simulink model "controlGPI_pos_6dof_sinMI"  (R2023b)
settings: Solver=ode45  StartTime=0.0  StopTime=tsim  FixedStep=tstep  MaxStep=tstep  RelTol=tstep/10
undefined symbols (not defined in the file): contr_robot_params, ddq, dq, ndof, NN_Bspline_params, NN_RBF_params, nn_select, Pc, q0, q_cero, q_eq, robot_params, t_qeq_init, t_tr_init, t_trtr, tau_L, tau_L_mags, tr_muestra, tr_ref, Wc, Zc
libraries: simulink x2
(part 2 of 2)

== system controlGPI_pos_6dof_sinMI/Trayectoria de referencia/3 to 9 (4) ==
  In1 : Inport
  In2 : Inport  Port=2
  In3 : Inport  Port=3
  Demux2 : Demux  Outputs=3
  Demux3 : Demux  Outputs=3
  Demux4 : Demux  Outputs=3
  Out1 : Outport
  Out2 : Outport  Port=2
  Out3 : Outport  Port=3
  Out4 : Outport  Port=4
  Out5 : Outport  Port=5
  Out6 : Outport  Port=6
  Out7 : Outport  Port=7
  Out8 : Outport  Port=8
  Out9 : Outport  Port=9
  wires:
  In3/1 -> Demux4/1
  Demux4/1 -> Out3/1
  Demux2/1 -> Out1/1
  Demux3/3 -> Out8/1
  Demux3/2 -> Out5/1
  Demux3/1 -> Out2/1
  In1/1 -> Demux2/1
  Demux2/3 -> Out7/1
  Demux4/3 -> Out9/1
  Demux4/2 -> Out6/1
  Demux2/2 -> Out4/1
  In2/1 -> Demux3/1

== system controlGPI_pos_6dof_sinMI/Trayectoria de referencia/3 to 9 (5) ==
  In1 : Inport
  In2 : Inport  Port=2
  In3 : Inport  Port=3
  Demux2 : Demux  Outputs=3
  Demux3 : Demux  Outputs=3
  Demux4 : Demux  Outputs=3
  Out1 : Outport
  Out2 : Outport  Port=2
  Out3 : Outport  Port=3
  Out4 : Outport  Port=4
  Out5 : Outport  Port=5
  Out6 : Outport  Port=6
  Out7 : Outport  Port=7
  Out8 : Outport  Port=8
  Out9 : Outport  Port=9
  wires:
  In3/1 -> Demux4/1
  Demux4/1 -> Out3/1
  Demux2/1 -> Out1/1
  Demux3/3 -> Out8/1
  Demux3/2 -> Out5/1
  Demux3/1 -> Out2/1
  In1/1 -> Demux2/1
  Demux2/3 -> Out7/1
  Demux4/3 -> Out9/1
  Demux4/2 -> Out6/1
  Demux2/2 -> Out4/1
  In2/1 -> Demux3/1

== system controlGPI_pos_6dof_sinMI/Trayectoria de referencia/3 to 9 (7) ==
  In1 : Inport
  In2 : Inport  Port=2
  In3 : Inport  Port=3
  Demux2 : Demux  Outputs=3
  Demux3 : Demux  Outputs=3
  Demux4 : Demux  Outputs=3
  Out1 : Outport
  Out2 : Outport  Port=2
  Out3 : Outport  Port=3
  Out4 : Outport  Port=4
  Out5 : Outport  Port=5
  Out6 : Outport  Port=6
  Out7 : Outport  Port=7
  Out8 : Outport  Port=8
  Out9 : Outport  Port=9
  wires:
  In3/1 -> Demux4/1
  Demux4/1 -> Out3/1
  Demux2/1 -> Out1/1
  Demux3/3 -> Out8/1
  Demux3/2 -> Out5/1
  Demux3/1 -> Out2/1
  In1/1 -> Demux2/1
  Demux2/3 -> Out7/1
  Demux4/3 -> Out9/1
  Demux4/2 -> Out6/1
  Demux2/2 -> Out4/1
  In2/1 -> Demux3/1

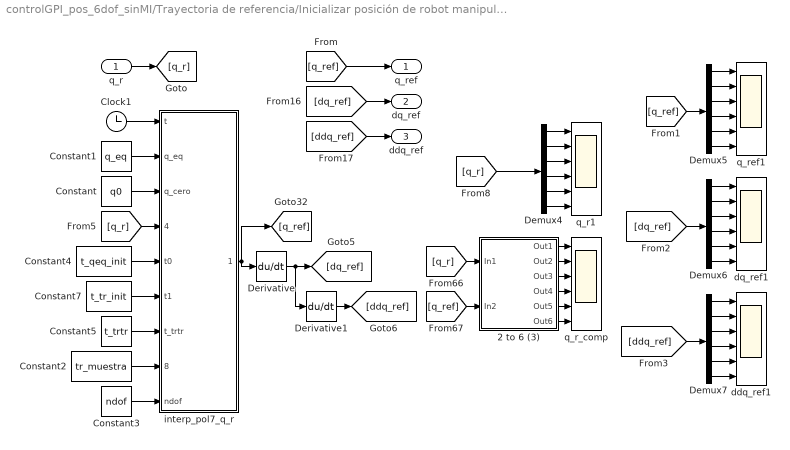
== system controlGPI_pos_6dof_sinMI/Trayectoria de referencia/Inicializar posición de robot manipulador ==
  q_r : Inport
  2 to 6 (3) : Subsystem
  Clock1 : Clock
  Constant : Constant  Value=q0
  Constant1 : Constant  Value=q_eq
  Constant2 : Constant  Value=tr_muestra
  Constant3 : Constant  Value=ndof
  Constant4 : Constant  Value=t_qeq_init
  Constant5 : Constant  Value=t_trtr
  Constant7 : Constant  Value=t_tr_init
  Demux{4..7} (4 alike) : Demux  Outputs=6
  Derivative : Derivative
  Derivative1 : Derivative
  ddq_ref1 : Scope  NumInputPorts=6
  dq_ref1 : Scope  NumInputPorts=6
  interp_pol7_q_r : MATLAB Function  TreatAsAtomicUnit=on
  q_r1 : Scope  NumInputPorts=6
  q_r_comp : Scope  NumInputPorts=6
  q_ref1 : Scope  NumInputPorts=6
  q_ref : Outport
  dq_ref : Outport  Port=2
  ddq_ref : Outport  Port=3
  wires:
  [ddq_ref] -> ddq_ref/1
  q_r/1 -> [q_r]
  [dq_ref] -> dq_ref/1
  [q_ref] -> q_ref/1
  2 to 6 (3)/1(Out1) -> q_r_comp/1
  [q_r] -> 2 to 6 (3)/1(In1)
  2 to 6 (3)/3(Out3) -> q_r_comp/3
  2 to 6 (3)/5(Out5) -> q_r_comp/5
  2 to 6 (3)/6(Out6) -> q_r_comp/6
  [q_ref] -> 2 to 6 (3)/2(In2)
  2 to 6 (3)/2(Out2) -> q_r_comp/2
  2 to 6 (3)/4(Out4) -> q_r_comp/4
  Demux4/3 -> q_r1/3
  Demux4/5 -> q_r1/5
  Demux4/4 -> q_r1/4
  Demux4/2 -> q_r1/2
  Demux4/6 -> q_r1/6
  Demux4/1 -> q_r1/1
  [q_r] -> Demux4/1
  Constant7/1 -> interp_pol7_q_r/6(t1)
  Clock1/1 -> interp_pol7_q_r/1(t)
  interp_pol7_q_r/1(interp_qpos) -> Derivative/1, [q_ref]
  Constant1/1 -> interp_pol7_q_r/2(q_eq)
  Constant/1 -> interp_pol7_q_r/3(q_cero)
  Derivative/1 -> [dq_ref], Derivative1/1
  Derivative1/1 -> [ddq_ref]
  Demux5/6 -> q_ref1/6
  Demux5/2 -> q_ref1/2
  [q_ref] -> Demux5/1
  Demux5/1 -> q_ref1/1
  Demux5/4 -> q_ref1/4
  Demux5/5 -> q_ref1/5
  Demux5/3 -> q_ref1/3
  Demux6/1 -> dq_ref1/1
  Demux6/4 -> dq_ref1/4
  Demux6/5 -> dq_ref1/5
  [dq_ref] -> Demux6/1
  Demux6/6 -> dq_ref1/6
  Demux6/2 -> dq_ref1/2
  Demux6/3 -> dq_ref1/3
  Demux7/2 -> ddq_ref1/2
  Demux7/4 -> ddq_ref1/4
  Demux7/3 -> ddq_ref1/3
  [ddq_ref] -> Demux7/1
  Demux7/1 -> ddq_ref1/1
  Demux7/6 -> ddq_ref1/6
  Demux7/5 -> ddq_ref1/5
  [q_r] -> interp_pol7_q_r/4(q_tr_init)
  Constant4/1 -> interp_pol7_q_r/5(t0)
  Constant2/1 -> interp_pol7_q_r/8(tr_muestra)
  Constant3/1 -> interp_pol7_q_r/9(ndof)
  Constant5/1 -> interp_pol7_q_r/7(t_trtr)

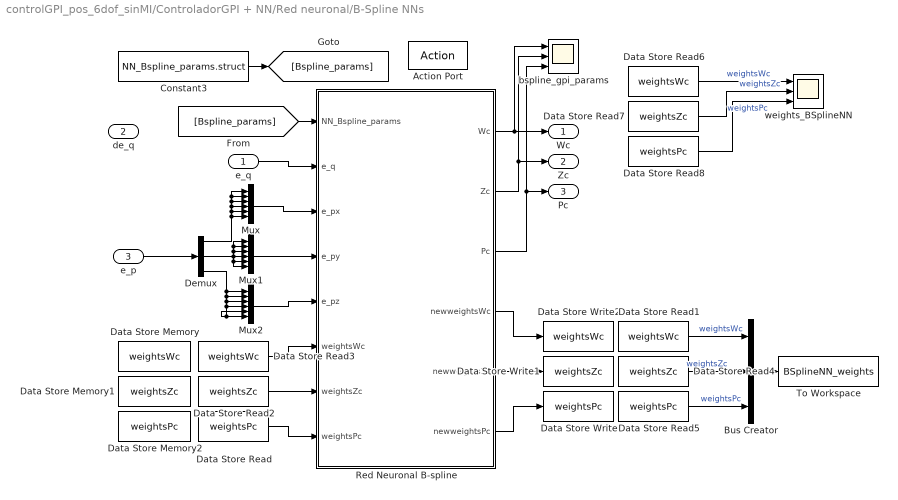
== system controlGPI_pos_6dof_sinMI/ControladorGPI + NN/Red neuronal/B-Spline NNs ==
  e_q : Inport
  de_q : Inport  Port=2
  e_p : Inport  Port=3
  Action Port : ActionPort  ActionPortLabel=if(u1 == 1)
  Bus Creator : BusCreator  Inputs=3
  Constant3 : Constant  Value=NN_Bspline_params.struct  OutDataTypeStr=Bus: NN_Bspline_params_bus
  Data Store Memory : DataStoreMemory  DataStoreName=weightsWc  WriteAfterWriteMsg=warning  InitialValue=NN_Bspline_params.weights.weightWc  ShowAdditionalParam=off  OutDataTypeStr=double
  Data Store Memory1 : DataStoreMemory  DataStoreName=weightsZc  WriteAfterWriteMsg=warning  InitialValue=NN_Bspline_params.weights.weightZc  ShowAdditionalParam=off  OutDataTypeStr=double
  Data Store Memory2 : DataStoreMemory  DataStoreName=weightsPc  WriteAfterWriteMsg=warning  InitialValue=NN_Bspline_params.weights.weightPc  ShowAdditionalParam=off  OutDataTypeStr=double
  Data Store Read : DataStoreRead  DataStoreName=weightsPc  IndexOptions=Index vector (dialog)  Indices=1  OutputSizes=1
  Data Store Read1 : DataStoreRead  DataStoreName=weightsWc  IndexOptions=Index vector (dialog)  Indices=1  OutputSizes=1
  Data Store Read2 : DataStoreRead  DataStoreName=weightsZc  IndexOptions=Index vector (dialog)  Indices=1  OutputSizes=1
  Data Store Read3 : DataStoreRead  DataStoreName=weightsWc  IndexOptions=Index vector (dialog)  Indices=1  OutputSizes=1
  Data Store Read4 : DataStoreRead  DataStoreName=weightsZc  IndexOptions=Index vector (dialog)  Indices=1  OutputSizes=1
  Data Store Read5 : DataStoreRead  DataStoreName=weightsPc  IndexOptions=Index vector (dialog)  Indices=1  OutputSizes=1
  Data Store Read6 : DataStoreRead  DataStoreName=weightsWc  IndexOptions=Index vector (dialog)  Indices=1  OutputSizes=1
  Data Store Read7 : DataStoreRead  DataStoreName=weightsZc  IndexOptions=Index vector (dialog)  Indices=1  OutputSizes=1
  Data Store Read8 : DataStoreRead  DataStoreName=weightsPc  IndexOptions=Index vector (dialog)  Indices=1  OutputSizes=1
  Data Store Write : DataStoreWrite  DataStoreName=weightsPc  IndexOptions=Index vector (dialog)  Indices=1  OutputSizes=1
  Data Store Write1 : DataStoreWrite  DataStoreName=weightsZc  IndexOptions=Index vector (dialog)  Indices=1  OutputSizes=1
  Data Store Write2 : DataStoreWrite  DataStoreName=weightsWc  IndexOptions=Index vector (dialog)  Indices=1  OutputSizes=1
  Demux : Demux  Outputs=3
  Mux : Mux  Inputs=6
  Mux1 : Mux  Inputs=6
  Mux2 : Mux  Inputs=6
  Red Neuronal B-spline : MATLAB Function  TreatAsAtomicUnit=on
  To Workspace : ToWorkspace  VariableName=BSplineNN_weights  SaveFormat=Timeseries  SampleTime=-1
  bspline_gpi_params : Scope  NumInputPorts=3
  weights_BSplineNN : Scope  NumInputPorts=3
  Wc : Outport
  Zc : Outport  Port=2
  Pc : Outport  Port=3
  wires:
  e_q/1 -> Red Neuronal B-spline/2(e_q)
  [Bspline_params] -> Red Neuronal B-spline/1(NN_Bspline_params)
  Red Neuronal B-spline/1(Wc) -> bspline_gpi_params/1, Wc/1
  Red Neuronal B-spline/2(Zc) -> bspline_gpi_params/2, Zc/1
  Red Neuronal B-spline/3(Pc) -> bspline_gpi_params/3, Pc/1
  Constant3/1 -> [Bspline_params]
  Data Store Read1/1 -> Bus Creator/1  "weightsWc"
  Data Store Read5/1 -> Bus Creator/3  "weightsPc"
  Bus Creator/1 -> To Workspace/1
  Data Store Read4/1 -> Bus Creator/2  "weightsZc"
  Red Neuronal B-spline/4(newweightsWc) -> Data Store Write2/1
  Red Neuronal B-spline/5(newweightsZc) -> Data Store Write1/1
  Red Neuronal B-spline/6(newweightsPc) -> Data Store Write/1
  Data Store Read3/1 -> Red Neuronal B-spline/6(weightsWc)
  Data Store Read2/1 -> Red Neuronal B-spline/7(weightsZc)
  Data Store Read/1 -> Red Neuronal B-spline/8(weightsPc)
  Data Store Read6/1 -> weights_BSplineNN/1  "weightsWc"
  Data Store Read7/1 -> weights_BSplineNN/2  "weightsZc"
  Data Store Read8/1 -> weights_BSplineNN/3  "weightsPc"
  e_p/1 -> Demux/1
  Demux/3 -> Mux2/3, Mux2/5, Mux2/6, Mux2/4, Mux2/2, Mux2/1
  Mux/1 -> Red Neuronal B-spline/3(e_px)
  Demux/1 -> Mux/6, Mux/5, Mux/4, Mux/3, Mux/1, Mux/2
  Mux2/1 -> Red Neuronal B-spline/5(e_pz)
  Demux/2 -> Mux1/6, Mux1/5, Mux1/4, Mux1/2, Mux1/1, Mux1/3
  Mux1/1 -> Red Neuronal B-spline/4(e_py)

== system controlGPI_pos_6dof_sinMI/ControladorGPI + NN/Red neuronal/Constants ==
  Action Port : ActionPort  ActionPortLabel=else
  Constant : Constant  Value=Wc
  Constant1 : Constant  Value=Zc
  Constant2 : Constant  Value=Pc
  Scope1 : Scope  NumInputPorts=3
  Wc : Outport
  Zc : Outport  Port=2
  Pc : Outport  Port=3
  wires:
  Constant/1 -> Wc/1, Scope1/1
  Constant2/1 -> Scope1/3, Pc/1
  Constant1/1 -> Zc/1, Scope1/2

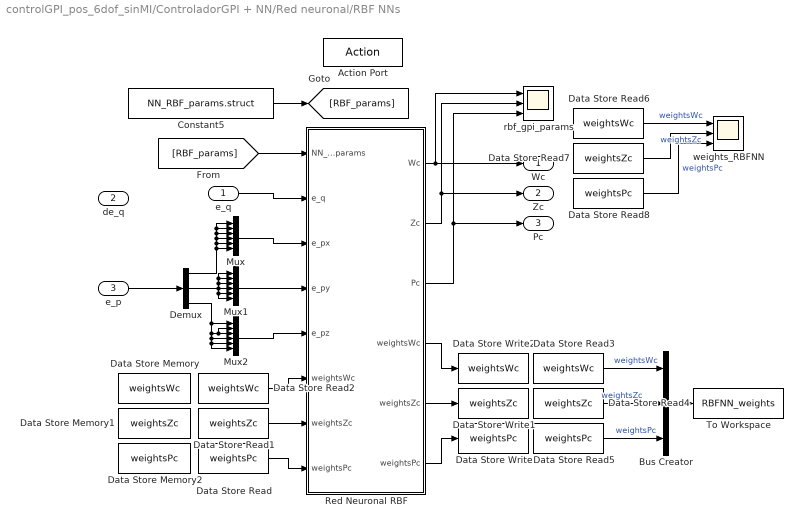
== system controlGPI_pos_6dof_sinMI/ControladorGPI + NN/Red neuronal/RBF NNs ==
  e_q : Inport
  de_q : Inport  Port=2
  e_p : Inport  Port=3
  Action Port : ActionPort  ActionPortLabel=elseif(u1 == 2)
  Bus Creator : BusCreator  Inputs=3
  Constant5 : Constant  Value=NN_RBF_params.struct  OutDataTypeStr=Bus: NN_RBF_params_bus
  Data Store Memory : DataStoreMemory  DataStoreName=weightsWc  WriteAfterWriteMsg=warning  InitialValue=NN_RBF_params.weights.weightWc  ShowAdditionalParam=off  OutDataTypeStr=double
  Data Store Memory1 : DataStoreMemory  DataStoreName=weightsZc  WriteAfterWriteMsg=warning  InitialValue=NN_RBF_params.weights.weightZc  ShowAdditionalParam=off  OutDataTypeStr=double
  Data Store Memory2 : DataStoreMemory  DataStoreName=weightsPc  WriteAfterWriteMsg=warning  InitialValue=NN_RBF_params.weights.weightPc  ShowAdditionalParam=off  OutDataTypeStr=double
  Data Store Read : DataStoreRead  DataStoreName=weightsPc  IndexOptions=Index vector (dialog)  Indices=1  OutputSizes=1
  Data Store Read1 : DataStoreRead  DataStoreName=weightsZc  IndexOptions=Index vector (dialog)  Indices=1  OutputSizes=1
  Data Store Read2 : DataStoreRead  DataStoreName=weightsWc  IndexOptions=Index vector (dialog)  Indices=1  OutputSizes=1
  Data Store Read3 : DataStoreRead  DataStoreName=weightsWc  IndexOptions=Index vector (dialog)  Indices=1  OutputSizes=1
  Data Store Read4 : DataStoreRead  DataStoreName=weightsZc  IndexOptions=Index vector (dialog)  Indices=1  OutputSizes=1
  Data Store Read5 : DataStoreRead  DataStoreName=weightsPc  IndexOptions=Index vector (dialog)  Indices=1  OutputSizes=1
  Data Store Read6 : DataStoreRead  DataStoreName=weightsWc  IndexOptions=Index vector (dialog)  Indices=1  OutputSizes=1
  Data Store Read7 : DataStoreRead  DataStoreName=weightsZc  IndexOptions=Index vector (dialog)  Indices=1  OutputSizes=1
  Data Store Read8 : DataStoreRead  DataStoreName=weightsPc  IndexOptions=Index vector (dialog)  Indices=1  OutputSizes=1
  Data Store Write : DataStoreWrite  DataStoreName=weightsPc  IndexOptions=Index vector (dialog)  Indices=1  OutputSizes=1
  Data Store Write1 : DataStoreWrite  DataStoreName=weightsZc  IndexOptions=Index vector (dialog)  Indices=1  OutputSizes=1
  Data Store Write2 : DataStoreWrite  DataStoreName=weightsWc  IndexOptions=Index vector (dialog)  Indices=1  OutputSizes=1
  Demux : Demux  Outputs=3
  Mux : Mux  Inputs=6
  Mux1 : Mux  Inputs=6
  Mux2 : Mux  Inputs=6
  Red Neuronal RBF : MATLAB Function  TreatAsAtomicUnit=on
  To Workspace : ToWorkspace  VariableName=RBFNN_weights  SaveFormat=Timeseries  SampleTime=-1
  rbf_gpi_params : Scope  NumInputPorts=3
  weights_RBFNN : Scope  NumInputPorts=3
  Wc : Outport
  Zc : Outport  Port=2
  Pc : Outport  Port=3
  wires:
  [RBF_params] -> Red Neuronal RBF/1(NN_RBF_params)
  e_q/1 -> Red Neuronal RBF/2(e_q)
  Red Neuronal RBF/1(Wc) -> rbf_gpi_params/1, Wc/1
  Red Neuronal RBF/2(Zc) -> rbf_gpi_params/2, Zc/1
  Red Neuronal RBF/3(Pc) -> rbf_gpi_params/3, Pc/1
  Data Store Read/1 -> Red Neuronal RBF/8("weightsPc ")
  Data Store Read1/1 -> Red Neuronal RBF/7("weightsZc ")
  Data Store Read2/1 -> Red Neuronal RBF/6("weightsWc ")
  Data Store Read3/1 -> Bus Creator/1  "weightsWc"
  Data Store Read4/1 -> Bus Creator/2  "weightsZc"
  Data Store Read5/1 -> Bus Creator/3  "weightsPc"
  Bus Creator/1 -> To Workspace/1
  Red Neuronal RBF/6(weightsPc) -> Data Store Write/1
  Red Neuronal RBF/4(weightsWc) -> Data Store Write2/1
  Red Neuronal RBF/5(weightsZc) -> Data Store Write1/1
  Data Store Read6/1 -> weights_RBFNN/1  "weightsWc"
  Data Store Read7/1 -> weights_RBFNN/2  "weightsZc"
  Data Store Read8/1 -> weights_RBFNN/3  "weightsPc"
  Constant5/1 -> [RBF_params]
  e_p/1 -> Demux/1
  Mux/1 -> Red Neuronal RBF/3(e_px)
  Mux1/1 -> Red Neuronal RBF/4(e_py)
  Demux/3 -> Mux2/6, Mux2/5, Mux2/4, Mux2/3, Mux2/2, Mux2/1
  Mux2/1 -> Red Neuronal RBF/5(e_pz)
  Demux/1 -> Mux/6, Mux/5, Mux/4, Mux/3, Mux/1, Mux/2
  Demux/2 -> Mux1/6, Mux1/5, Mux1/4, Mux1/2, Mux1/1, Mux1/3

== system controlGPI_pos_6dof_sinMI/Trayectoria de referencia/Inicializar posición de robot manipulador/2 to 6 (3) ==
  In1 : Inport
  In2 : Inport  Port=2
  Demux4 : Demux  Outputs=6
  Demux6 : Demux  Outputs=6
  Mux{,1..5} (6 alike) : Mux  Inputs=2
  Out1 : Outport
  Out2 : Outport  Port=2
  Out3 : Outport  Port=3
  Out4 : Outport  Port=4
  Out5 : Outport  Port=5
  Out6 : Outport  Port=6
  wires:
  In2/1 -> Demux6/1
  Demux4/3 -> Mux2/1
  Demux4/5 -> Mux4/1
  Demux4/6 -> Mux5/1
  Demux6/5 -> Mux4/2
  Demux4/1 -> Mux/1
  Demux6/6 -> Mux5/2
  In1/1 -> Demux4/1
  Demux4/4 -> Mux3/1
  Demux6/2 -> Mux1/2
  Demux6/4 -> Mux3/2
  Demux6/1 -> Mux/2
  Demux4/2 -> Mux1/1
  Demux6/3 -> Mux2/2
  Mux/1 -> Out1/1
  Mux1/1 -> Out2/1
  Mux2/1 -> Out3/1
  Mux3/1 -> Out4/1
  Mux4/1 -> Out5/1
  Mux5/1 -> Out6/1

== matlab function controlGPI_pos_6dof_sinMI/ControladorGPI + NN/Matriz de parámetros B ==
  data: B5 output size=[6,1]; B4 output size=[6,1]; B3 output size=[6,1]; B2 output size=[6,1]; Zc input size=[6,1]; B1 output size=[6,1]; Wc input size=[6,1]; Pc input size=[6,1]
function [B5,B4,B3,B2,B1] = fcn(Zc,Wc,Pc)

B = zeros(6,6);

B(:,1) = Wc.^4.*Pc;
B(:,2) = 4*Wc.^3.*Zc.*Pc + Wc.^4;
B(:,3) = 4*Wc.^3.*Zc + 4*Wc.^2.*Zc.^2.*Pc + 2.*Wc.^2.*Pc;
B(:,4) = 2*Wc.^2 + 4*Wc.^2.*Zc.^2 + 4*Wc.*Zc.*Pc;
B(:,5) = 4*Wc.*Zc + Pc;
% B(:,6) = ones(3,6);

B1 = B(:,1);
B2 = B(:,2);
B3 = B(:,3);
B4 = B(:,4);
B5 = B(:,5);
% B6 = B(:,6);

== matlab function controlGPI_pos_6dof_sinMI/ControladorGPI + NN/Red neuronal/B-Spline NNs/Red Neuronal B-spline ==
  data: NN_Bspline_params input; e_q input size=[6,1]; Wc output size=[6,1]; Zc output size=[6,1]; Pc output size=[6,1]; e_px input size=[6,1]; e_py input size=[6,1]; e_pz input size=[6,1]; newweightsWc output; newweightsZc output; newweightsPc output; weightsWc input; weightsZc input; weightsPc input
function [Wc, Zc, Pc, newweightsWc, newweightsZc, newweightsPc]   = BSpline_NN(NN_Bspline_params,e_q,e_px,e_py,e_pz,weightsWc,weightsZc,weightsPc)

deltaWc = NN_Bspline_params.delta.deltaWc;
deltaZc = NN_Bspline_params.delta.deltaZc;
deltaPc = NN_Bspline_params.delta.deltaPc;

lambdaWc = NN_Bspline_params.lambda.lambdaWc;
lambdaZc = NN_Bspline_params.lambda.lambdaZc;
lambdaPc = NN_Bspline_params.lambda.lambdaPc;

if NN_Bspline_params.num_inputs == 1
    nn_inputs = e_q;
elseif NN_Bspline_params.num_inputs == 4
    nn_inputs = [e_q,e_px,e_py,e_pz];
else
    nn_inputs = e_q;
end

delta = [deltaWc;
         deltaZc;
         deltaPc];

lambda = cat(1,lambdaWc,lambdaZc,lambdaPc);
weights = cat(1,weightsWc,weightsZc,weightsPc);

[newparams,newweights] = NN_Bspline.Gradient_Descent(delta,weights,lambda,nn_inputs);

Wc = newparams(1,:)';
Zc = newparams(2,:)';
Pc = newparams(3,:)';

newweightsWc = newweights(1,:,:);
newweightsZc = newweights(2,:,:);
newweightsPc = newweights(3,:,:);

end

== matlab function controlGPI_pos_6dof_sinMI/Perfil torque de carga tau_L/If Action Subsystem/Polinomio 7mo orden sen ==
  data: t input; perfil_params input; qpol output; vpol output; apol output; jpol output
function [qpol,vpol,apol,jpol] = fcn(t,perfil_params)

%Trayectoria de referencia

q0 = 0;
q1 = perfil_params.senoidal.amplitud;

% v0 = perfil_params.polinomio7.vel.inicial;
% v1 = perfil_params.polinomio7.vel.final;
% 
% ac0 = perfil_params.polinomio7.acel.inicial;
% ac1 = perfil_params.polinomio7.acel.final;
% 
% j0 = perfil_params.polinomio7.jerk.inicial;
% j1 = perfil_params.polinomio7.jerk.inicial;

if perfil_params.senoidal.tiempo_inicio-1>0
    t0 = perfil_params.senoidal.tiempo_inicio-1;
else
    t0 = 0;
end
t1 = perfil_params.senoidal.tiempo_inicio;

% Coeficientes de un polinomio de 7mo grado
[qpol,vpol,apol,jpol] = pol7(t,q1,q0,t0,t1);

== matlab function controlGPI_pos_6dof_sinMI/Perfil torque de carga tau_L/If Action Subsystem4/Polinomio 7mo orden tau_L ==
  data: t input; perfil_params input; qpol output; vpol output; apol output; jpol output
function [qpol,vpol,apol,jpol] = fcn(t,perfil_params)

%Trayectoria de referencia

q0 = perfil_params.polinomio7.pos.inicial;
q1 = perfil_params.polinomio7.pos.final;

% v0 = perfil_params.polinomio7.vel.inicial;
% v1 = perfil_params.polinomio7.vel.final;
% 
% ac0 = perfil_params.polinomio7.acel.inicial;
% ac1 = perfil_params.polinomio7.acel.final;
% 
% j0 = perfil_params.polinomio7.jerk.inicial;
% j1 = perfil_params.polinomio7.jerk.inicial;

t0 = perfil_params.polinomio7.tiempo.inicial;
t1 = perfil_params.polinomio7.tiempo.final;

% Coeficientes de un polinomio de 7mo grado
[qpol,vpol,apol,jpol] = pol7(t,q0,q1,t0,t1);

== matlab function controlGPI_pos_6dof_sinMI/Perfil torque de carga tau_L/If Action Subsystem7/Trayectoria 15 segmentos ==
  data: t input size=1; q output size=1; perfil_params input
function q = fcn(t,perfil_params)

q0 = perfil_params.tr15segs.pos.inicial;
q1 = perfil_params.tr15segs.pos.final;

t0 = perfil_params.tr15segs.tiempo.inicial;

vel_path = perfil_params.tr15segs.vel_path;
acel_path = perfil_params.tr15segs.acel_path;
snap_path = perfil_params.tr15segs.snap_path;

dist = norm(q1-q0);
num_steps = 1000;




[interq,T] = pol15segs.bounded_tr(dist,num_steps,vel_path,acel_path,snap_path,0);

tstep = T/num_steps;
t1 = t0 + T;
t_tr = (t0:tstep:t1)';


[~,idt] = min(t_tr-t);
dire = (q1 - q0)/dist;
q = q0 + dire*interq(idt);

== matlab function controlGPI_pos_6dof_sinMI/ISCI ==
  data: tau input; ISCI output
function ISCI = fcn(tau)

ISCI = tau.^2;

== matlab function controlGPI_pos_6dof_sinMI/Perfil torque de carga tau_L/If Action Subsystem6/Polinomio 7mo orden timeseries ==
  data: t input; qpol output; vpol output; apol output; jpol output
function [qpol,vpol,apol,jpol] = fcn(t)

q0 = 0;
q1 = 1;

t0 = 0.5;
t1 = 1;

%Trayectoria de referencia

% Coeficientes de un polinomio de 7mo grado
[qpol,vpol,apol,jpol] = pol7(t,q0,q1,t0,t1);

== matlab function controlGPI_pos_6dof_sinMI/Perfil torque de carga tau_L/If Action Subsystem/Senoidal tiempo de inicio ==
  data: t input; tr output; perfil_params input
function tr = fcn(t,perfil_params)

t1 = perfil_params.senoidal.tiempo_inicio;

if t < t1
    tr = 0;
else
    tr = t - t1;
end

== matlab function controlGPI_pos_6dof_sinMI/Perfil torque de carga tau_L/If Action Subsystem5/Tren de esca ==
  data: t input; q output; perfil_params input
function q = fcn(t,perfil_params)

q = Perfil_trayectoria.trEsca(t,perfil_params);

== matlab function controlGPI_pos_6dof_sinMI/ITAE ==
  data: t input; ITAE output; eq input
function ITAE = fcn(t,eq)

ITAE = t.*abs(eq);

== matlab function controlGPI_pos_6dof_sinMI/Modelo robot manipulador (Dinámica directa)/Dinámica directa ==
  data: robot_params input; q input; ddq output size=[6,1]; dq input size=[6,1]; tau_R input size=[6,1]; tau_L input size=[6,1]
function ddq = fcn(robot_params,q,dq,tau_R,tau_L)

robot_din = robot_dinm.din_6dof(robot_params,q,dq);

D = robot_din.D;
C = robot_din.C;
G = robot_din.G;
g = robot_din.g;

ddq = D^-1*(-C*dq-G*g+(tau_R-tau_L));

== matlab function controlGPI_pos_6dof_sinMI/Trayectoria de referencia/Dinamica inversa (referencia) ==
  data: robot_params input; tau_s output size=[6,1]; q input size=[6,1]; dq input size=[6,1]; ddq input size=[6,1]
function tau_s = fcn(robot_params,q,dq,ddq)

robot_din = robot_dinm.din_6dof(robot_params,q,dq);

D = robot_din.D;
C = robot_din.C;
G = robot_din.G;
g = robot_din.g;

tau_s = D*ddq + C*dq + G*g;

== matlab function controlGPI_pos_6dof_sinMI/Trayectoria de referencia/q to xyz (referencia) ==
  data: p output size=[3,6]; robot_params input; q input size=[6,1]; dq input; ddq input; dp output; ddp output
function [p,dp,ddp] = fcn(robot_params,q,dq,ddq)

[p,dp,ddp] = robot_cin.cin_dir_6dof(robot_params,q,dq,ddq);

== matlab function controlGPI_pos_6dof_sinMI/Trayectoria de referencia/xyz to q (referencia) ==
  data: robot_params input; q output size=[6,1]; r input size=[3,1]; dr input size=[3,1]; ddr input size=[3,1]; dq output size=[6,1]; ddq output size=[6,1]; R input size=[3,3]
function [q,dq,ddq] = fcn(robot_params,r,dr,ddr,R)

[q,dq,ddq] = robot_cin.cin_inv_6dof(robot_params,r,dr,ddr,R);

== matlab function controlGPI_pos_6dof_sinMI/ControladorGPI + NN/Matriz D ==
  data: robot_params input Bus: robot_params_bus; robot_din output Bus: robot_din_bus; q input
function robot_din = fcn(robot_params,q)

robot_din = robot_dinm.din_6dof(robot_params,q,zeros(size(q)));

== matlab function controlGPI_pos_6dof_sinMI/q to xyz (robot)/q to xyz (robot) ==
  data: p output size=[3,6]; robot_params input; q input size=[6,1]; dq input size=[6,1]; ddq input size=[6,1]; dp output size=[3,1]; ddp output size=[3,1]
function [p,dp,ddp] = fcn(robot_params,q,dq,ddq)

p = robot_cin.cin_dirp_6dof(robot_params,q);

JP = robot_cin.JP_6dof(robot_params,q);
dp = JP*dq;

dJP = robot_cin.dJP_6dof(robot_params,q,dq);
ddp = dJP*ddq;

== matlab function controlGPI_pos_6dof_sinMI/ControladorGPI + NN/Red neuronal/RBF NNs/Red Neuronal RBF ==
  data: NN_RBF_params input; e_q input size=[6,1]; Wc output size=[6,1]; Zc output size=[6,1]; Pc output size=[6,1]; e_px input size=[6,1]; e_py input size=[6,1]; e_pz input size=[6,1]; weightsWc output; weightsZc output; weightsPc output; weightsWc input; weightsZc input; weightsPc input
function [Wc, Zc, Pc, weightsWc, weightsZc, weightsPc] = RBF_NN(NN_RBF_params,e_q,e_px,e_py,e_pz, weightsWc, weightsZc, weightsPc)

%k = NN_RBF_params.rbf_params.k;
centers = NN_RBF_params.rbf_params.C';
radius = NN_RBF_params.rbf_params.sigma;

deltaWc = NN_RBF_params.delta.deltaWc;
deltaZc = NN_RBF_params.delta.deltaZc;
deltaPc = NN_RBF_params.delta.deltaPc;

if NN_RBF_params.num_inputs == 1
    NNRBF_inputs = e_q;
elseif NN_RBF_params.num_inputs == 4
    NNRBF_inputs = [e_q,e_px,e_py,e_pz];
else
    NNRBF_inputs = e_q;
end

delta = [deltaWc;
         deltaZc;
         deltaPc];

weights = cat(1,weightsWc,weightsZc,weightsPc);

[newparams,newweights] = NN_RBF.Gradient_Descent(delta,weights,centers,radius,NNRBF_inputs);

Wc = newparams(1,:)';
Zc = newparams(2,:)';
Pc = newparams(3,:)';

weightsWc = newweights(1,:,:);
weightsZc = newweights(2,:,:);
weightsPc = newweights(3,:,:);

end

== matlab function controlGPI_pos_6dof_sinMI/Trayectoria de referencia/Inicializar posición de robot manipulador/interp_pol7_q_r ==
  data: t input; q_eq input; interp_qpos output; q_cero input; q_tr_init input; t0 input; t1 input; t_trtr input; tr_muestra input; ndof input
function interp_qpos = fcn(t,q_eq,q_cero,q_tr_init,t0,t1,t_trtr,tr_muestra,ndof)

tcero = t0/2 + t1/2;

if t < tcero
    dist1 = norm(zeros(size(q_eq)) - q_eq);
    
    if dist1 > 0
        qpol1 = pol7(t,0,dist1,t0,tcero);
        dire1 = (zeros(size(q_eq)) - q_eq)/dist1;
        
        interp_qpos = q_eq + dire1*qpol1;
    else
        interp_qpos = q_eq;
    end
elseif t >= tcero && t < t1
    dist2 = norm(q_cero - zeros(size(q_eq)));
    if dist2 > 0
        qpol2 = pol7(t,0,dist2,tcero,t1);
        dire2 = (q_cero - zeros(size(q_eq)))/dist2;
    
        interp_qpos =  zeros(size(q_eq)) + dire2*qpol2;
    else
        interp_qpos = zeros(size(q_eq));
    end
elseif t >= t1 && t < t1 + t_trtr
    if (tr_muestra == 1 || ndof ~= 6) && ndof ~= 2
        dist3 = norm(q_tr_init - q_cero);
        if dist3 > 0
            qpol3 = pol7(t,0,dist3,t1,t1 + t_trtr);
            dire3 = (q_tr_init - q_cero)/dist3;
            
            interp_qpos =  q_cero + dire3*qpol3;
        else
            interp_qpos = q_cero;
        end
    else
        interp_qpos = q_tr_init;
    end
elseif t >= t1 + t_trtr
    interp_qpos = q_tr_init;
else
    interp_qpos = q_eq;
end

== matlab function controlGPI_pos_6dof_sinMI/Norm e_q ==
  data: u input; y output
function y = norm(u)

y = norm(u,2);

== matlab function controlGPI_pos_6dof_sinMI/ControladorGPI + NN/Ley de control ==
  data: robot_din input; v output size=[6,1]; eqB5 input size=[6,1]; eqB4 input size=[6,1]; eqB3 input size=[6,1]; eqB2 input size=[6,1]; eqB1 input size=[6,1]; tau_R output size=[6,1]
function [v,tau_R] = fcn(robot_din,eqB5,eqB4,eqB3,eqB2,eqB1)

D = robot_din.D;

v = - eqB5 - eqB4 - eqB3 - eqB2 - eqB1;

tau_R = D*v;
